simulink model "jerkControl2017"  (Simulink 8.9)
settings: Solver=FixedStepDiscrete  StartTime=0.0  StopTime="Config.SIMULATION_TIME "  FixedStep=Config.Ts  RelTol=1e-3  EnableMultiTasking=on
InitFcn:
  | %% initialize the simulation
  | cd(fileparts(which(bdroot)));
  | initJerkControl;
StopFcn:
  | %% stop the simulation
  | cd(fileparts(which(bdroot)));
  | stopJerkControl;
undefined symbols (not defined in the file or in its folder): Config, DiscIntNeverNeededParam, Gain, Reg, ROBOT_DOF, Sat, Sm
libraries: WBToolboxLibrary x69, simulink x4
(part 2 of 2)

== system jerkControl2017/emergency stop: joint limits/STOP IF THERE ARE SPIKES IN THE ENCODERS ==
  qj : Inport
  Enable : EnablePort
  Assertion : Assertion
  MATLAB Function : MATLAB Function  TreatAsAtomicUnit=on
  index1 : Constant  Value=Sat.maxJointsPositionDelta  VectorParams1D=off
  wires:
  qj/1 -> MATLAB Function/1(u)
  MATLAB Function/1(noSpikes) -> Assertion/1
  index1/1 -> MATLAB Function/2(delta_u_max)

== system jerkControl2017/synchronizer/GAZEBO_SYNCHRONIZER ==
  Enable : EnablePort
  Simulator Synchronizer : WBToolboxLibrary/Utilities/Simulator Synchronizer  period=Config.Ts  serverPortName='/clock/rpc'  clientPortName='/WBT_synchronizer/rpc:o'
      settings: SourceProductName=WholeBodyToolbox

== system jerkControl2017/synchronizer/REAL_TIME_SYNC ==
  Enable : EnablePort
  Real Time Synchronizer : WBToolboxLibrary/Utilities/Real Time Synchronizer  period=Config.Ts
      settings: SourceProductName=WholeBodyToolbox

== system jerkControl2017/Dump and visualize/Visualizer Forces and Momentum/dynamics_measured ==
  error : Inport
  Demux19 : Demux  Outputs=[3;3]
  Demux23 : Demux  Outputs=[6;6]
  Demux24 : Demux  Outputs=[3;3]
  left foot error wrench : Scope  NumInputPorts=2
  right foot error wrench : Scope  NumInputPorts=2
  wires:
  Demux19/2 -> right foot error wrench/2  "moments"
  Demux24/1 -> left foot error wrench/1  "forces"
  Demux24/2 -> left foot error wrench/2  "moments"
  Demux23/1 -> Demux24/1
  error/1 -> Demux23/1
  Demux19/1 -> right foot error wrench/1  "forces"
  Demux23/2 -> Demux19/1

== system jerkControl2017/Dump and visualize/Visualizer Forces and Momentum/star_dynamics ==
  error : Inport
  Demux19 : Demux  Outputs=[3;3]
  Demux23 : Demux  Outputs=[6;6]
  Demux24 : Demux  Outputs=[3;3]
  left foot error wrench : Scope  NumInputPorts=2
  right foot error wrench : Scope  NumInputPorts=2
  wires:
  Demux23/1 -> Demux24/1
  Demux19/1 -> right foot error wrench/1  "forces"
  Demux23/2 -> Demux19/1
  Demux19/2 -> right foot error wrench/2  "moments"
  Demux24/2 -> left foot error wrench/2  "moments"
  error/1 -> Demux23/1
  Demux24/1 -> left foot error wrench/1  "forces"

== system jerkControl2017/Dump and visualize/Visualizer Forces and Momentum/star_measured ==
  error : Inport
  Demux19 : Demux  Outputs=[3;3]
  Demux23 : Demux  Outputs=[6;6]
  Demux24 : Demux  Outputs=[3;3]
  left foot error wrench : Scope  NumInputPorts=2
  right foot error wrench : Scope  NumInputPorts=2
  wires:
  Demux19/2 -> right foot error wrench/2  "moments"
  Demux24/1 -> left foot error wrench/1  "forces"
  Demux24/2 -> left foot error wrench/2  "moments"
  Demux23/1 -> Demux24/1
  error/1 -> Demux23/1
  Demux19/1 -> right foot error wrench/1  "forces"
  Demux23/2 -> Demux19/1

== system jerkControl2017/Dynamics and Kinematics/Dynamics/Add motors reflected inertia ==
  M : Inport
  Add motor reflected inertias : MATLAB Function  TreatAsAtomicUnit=on
  Constant : Constant  Value=Config.USE_MOTOR_REFLECTED_INERTIA
  Switch : Switch  Criteria=u2 > Threshold
  M_with_motor_inertia : Outport
  wires:
  M/1 -> Switch/3, Add motor reflected inertias/1(M)
  Constant/1 -> Switch/2
  Add motor reflected inertias/1(M_with_inertia) -> Switch/1
  Switch/1 -> M_with_motor_inertia/1

== system jerkControl2017/Dynamics and Kinematics/Kinematics/xCom ==
  w_H_b : Inport
  qj : Inport  Port=2
  CoM : WBToolboxLibrary/Model/Kinematics/ForwardKinematics  frameName=Frames.COM
      settings: SourceProductName=WholeBodyToolbox
  "CoM6D ->  CoMXYZ2" : Selector  NumberOfDimensions=2  InputPortWidth=7  IndexOptions=Index vector (dialog),Index vector (dialog)  Indices=[1 2 3],[4]  OutputSizes=1,1
  xCoM : Outport
  wires:
  qj/1 -> CoM/2
  "CoM6D ->  CoMXYZ2"/1 -> xCoM/1
  CoM/1 -> "CoM6D ->  CoMXYZ2"/1
  w_H_b/1 -> CoM/1

== system jerkControl2017/Jerk Control/Compute angular momentum integral error (YOGA)/Compute base to fixed link transform ==
  jointPos : Inport
  Constant7 : Constant  Value=eye(4)
  "inv  " : Product  Inputs=/  Multiplication=Matrix(*)
  inv  1 : Product  Inputs=/  Multiplication=Matrix(*)
  l_sole to root_link relative transform : WBToolboxLibrary/Model/Kinematics/ForwardKinematics  frameName=Frames.LEFT_FOOT
      settings: SourceProductName=WholeBodyToolbox
  r_sole to root_link relative transform : WBToolboxLibrary/Model/Kinematics/ForwardKinematics  frameName=Frames.RIGHT_FOOT
      settings: SourceProductName=WholeBodyToolbox
  fixed_l_sole_H_b : Outport
  fixed_r_sole_H_b : Outport  Port=2
  wires:
  Constant7/1 -> l_sole to root_link relative transform/1, r_sole to root_link relative transform/1
  inv  1/1 -> fixed_r_sole_H_b/1
  "inv  "/1 -> fixed_l_sole_H_b/1
  jointPos/1 -> r_sole to root_link relative transform/2, l_sole to root_link relative transform/2
  l_sole to root_link relative transform/1 -> "inv  "/1
  r_sole to root_link relative transform/1 -> inv  1/1

== system jerkControl2017/Jerk Control/Estimate Contact Forces and Parametrization/From body to Mixed Representation ==
  w_H_l_sole : Inport
  w_H_r_sole : Inport  Port=2
  contactForces_wbd : Inport  Port=3
  MATLAB Function : MATLAB Function  TreatAsAtomicUnit=on
  contactForces_est : Outport
  wires:
  w_H_l_sole/1 -> MATLAB Function/1(w_H_l_sole)
  w_H_r_sole/1 -> MATLAB Function/2(w_H_r_sole)
  contactForces_wbd/1 -> MATLAB Function/3(f_body)
  MATLAB Function/1(f_mixed) -> contactForces_est/1

== system jerkControl2017/Jerk Control/Estimate Contact Forces and Parametrization/Get Parametrization from Forces ==
  LEFT_RIGHT_FOOT_IN_CONTACT : Inport
  contactForces_est : Inport  Port=2
  Constant : Constant  Value=[0;0;Config.fZmin;0;0;0]
  Constant1 : Constant  Value=[0;0;Config.fZmin;0;0;0]
  Demux : Demux  Outputs=[6;6]
  Demux1 : Demux  Outputs=[1;1]
  MATLAB Function1 : MATLAB Function  TreatAsAtomicUnit=on
  MATLAB Function2 : MATLAB Function  TreatAsAtomicUnit=on
  MatrixMultiply : Product
  MatrixMultiply1 : Product
  Mux : Mux  Inputs=2
  Switch : Switch  Criteria=u2 > Threshold
  Switch1 : Switch  Criteria=u2 > Threshold
  xi : Outport
  tag scope: xi_LFoot=global, xi_RFoot=global
  wires:
  Mux/1 -> xi/1
  contactForces_est/1 -> Demux/1
  LEFT_RIGHT_FOOT_IN_CONTACT/1 -> Demux1/1
  MATLAB Function1/1(xi) -> MatrixMultiply1/1
  MATLAB Function2/1(xi) -> MatrixMultiply/1
  Demux1/1 -> Switch/2, MatrixMultiply1/2
  Demux1/2 -> Switch1/2, MatrixMultiply/2
  MatrixMultiply1/1 -> Mux/1, [xi_LFoot]
  MatrixMultiply/1 -> Mux/2, [xi_RFoot]
  Demux/1 -> Switch/1
  Constant/1 -> Switch/3
  Demux/2 -> Switch1/1
  Constant1/1 -> Switch1/3
  Switch1/1 -> MATLAB Function2/1(contactForces)
  Switch/1 -> MATLAB Function1/1(contactForces)

== system jerkControl2017/Jerk Control/Integrate the Input Contact Forces Param. Derivative/Demux xiDot ==
  xiDot_star : Inport
  LEFT_RIGHT_FOOT_IN_CONTACT : Inport  Port=2
  M : Inport  Port=3
  Compute Initial Conditions LFoot : Subsystem
  Compute Initial Conditions RFoot : Subsystem
  Demux : Demux  Outputs=[6;6]
  Demux1 : Demux  Outputs=[1;1]
  MATLAB Function1 : MATLAB Function  TreatAsAtomicUnit=on
  MATLAB Function2 : MATLAB Function  TreatAsAtomicUnit=on
  xiDot_LFoot : Outport
  LFootContactActivation : Outport  Port=2
  init_xi_LFoot : Outport  Port=3
  xiDot_RFoot : Outport  Port=4
  RFootContactActivation : Outport  Port=5
  init_xi_RFoot : Outport  Port=6
  wires:
  Demux/2 -> xiDot_RFoot/1
  xiDot_star/1 -> Demux/1
  LEFT_RIGHT_FOOT_IN_CONTACT/1 -> Demux1/1
  Demux/1 -> xiDot_LFoot/1
  Demux1/1 -> Compute Initial Conditions LFoot/1(FOOT_IS_IN_CONTACT), LFootContactActivation/1
  Demux1/2 -> Compute Initial Conditions RFoot/1(FOOT_IS_IN_CONTACT), RFootContactActivation/1
  M/1 -> Compute Initial Conditions RFoot/2(M), Compute Initial Conditions LFoot/2(M)
  Compute Initial Conditions LFoot/1(contactForcesOneFoot_0) -> MATLAB Function1/1(contactForces)
  Compute Initial Conditions RFoot/1(contactForcesOneFoot_0) -> MATLAB Function2/1(contactForces)
  MATLAB Function1/1(xi) -> init_xi_LFoot/1
  MATLAB Function2/1(xi) -> init_xi_RFoot/1

== system jerkControl2017/Jerk Control/Integrate the Input Contact Forces Param. Derivative/From Parametrization to Forces ==
  LFootContactActivation : Inport
  xi_LFoot : Inport  Port=2
  xi_RFoot : Inport  Port=3
  RFootContactActivation : Inport  Port=4
  MATLAB Function : MATLAB Function  TreatAsAtomicUnit=on
  MATLAB Function1 : MATLAB Function  TreatAsAtomicUnit=on
  MatrixMultiply1 : Product
  MatrixMultiply2 : Product
  contactForces_LFoot : Outport
  contactForces_RFoot : Outport  Port=2
  wires:
  MatrixMultiply1/1 -> contactForces_LFoot/1
  MATLAB Function/1(contactForces) -> MatrixMultiply1/2
  MATLAB Function1/1(contactForces) -> MatrixMultiply2/2
  MatrixMultiply2/1 -> contactForces_RFoot/1
  LFootContactActivation/1 -> MatrixMultiply1/1
  xi_LFoot/1 -> MATLAB Function/1(xi)
  RFootContactActivation/1 -> MatrixMultiply2/1
  xi_RFoot/1 -> MATLAB Function1/1(xi)

== system jerkControl2017/Jerk Control/Integrate the Input Contact Forces Param. Derivative/deadZone ==
  u : Inport
  Constant : Constant  Value=Sat.deadZoneThreshold
  MATLAB Function : MATLAB Function  TreatAsAtomicUnit=on
  u_cut : Outport
  wires:
  MATLAB Function/1(y) -> u_cut/1
  u/1 -> MATLAB Function/1(u)
  Constant/1 -> MATLAB Function/2(thr)

== system jerkControl2017/Robot State and References/Internal Coordinator/Base to fixed_link ==
  qj : Inport
  inertial : Inport  Port=2
  Constant1 : Constant  Value=Config.LEFT_FOOT_IN_CONTACT_AT_0
  Constant7 : Constant  Value=eye(4)
  LFoot to world transform (fixed base) : WBToolboxLibrary/Model/Kinematics/ForwardKinematics  frameName=Frames.LEFT_FOOT
      settings: SourceProductName=WholeBodyToolbox
  RFoot to world transform (fixed base) : WBToolboxLibrary/Model/Kinematics/ForwardKinematics  frameName=Frames.RIGHT_FOOT
      settings: SourceProductName=WholeBodyToolbox
  Switch : Switch  Criteria=u2 > Threshold
  "fixedFoot to base link transform " : Subsystem
  fixed_LFoot_H_b : Outport
  wires:
  "fixedFoot to base link transform "/1(link_H_b) -> fixed_LFoot_H_b/1
  inertial/1 -> "fixedFoot to base link transform "/2(inertial)
  qj/1 -> "fixedFoot to base link transform "/1(qj), RFoot to world transform (fixed base)/2, LFoot to world transform (fixed base)/2
  Constant7/1 -> LFoot to world transform (fixed base)/1, RFoot to world transform (fixed base)/1, "fixedFoot to base link transform "/4(w_H_base_fixed)
  Switch/1 -> "fixedFoot to base link transform "/3(w_H_link)
  LFoot to world transform (fixed base)/1 -> Switch/1
  RFoot to world transform (fixed base)/1 -> Switch/3
  Constant1/1 -> Switch/2

== system jerkControl2017/Robot State and References/Internal Coordinator/Compute State Velocity ==
  qj : Inport
  w_H_b : Inport  Port=2
  "feetInContact " : Inport  Port=3
  Compute Base Velocity : MATLAB Function  TreatAsAtomicUnit=on
  Feet Jacobians : Subsystem
  GetMeasurement : WBToolboxLibrary/States/GetMeasurement  measuredType=Joints Velocity
      settings: SourceProductName=WholeBodyToolbox
  Mux : Mux  Inputs=2
  nu : Outport
  wires:
  GetMeasurement/1 -> Mux/2, Compute Base Velocity/4(jointVel)
  Mux/1 -> nu/1
  "feetInContact "/1 -> Compute Base Velocity/3(feetContactStatus)
  qj/1 -> Feet Jacobians/1(qj)
  w_H_b/1 -> Feet Jacobians/2(w_H_b)
  Feet Jacobians/1(J_LFoot) -> Compute Base Velocity/1(J_l_sole)
  Feet Jacobians/2(J_RFoot) -> Compute Base Velocity/2(J_r_sole)
  Compute Base Velocity/1(nu_b) -> Mux/1

== system jerkControl2017/Robot State and References/Internal Coordinator/xCom ==
  w_H_b : Inport
  qj : Inport  Port=2
  CoM : WBToolboxLibrary/Model/Kinematics/ForwardKinematics  frameName=Frames.COM
      settings: SourceProductName=WholeBodyToolbox
  "CoM6D ->  CoMXYZ2" : Selector  NumberOfDimensions=2  InputPortWidth=7  IndexOptions=Index vector (dialog),Index vector (dialog)  Indices=[1 2 3],[4]  OutputSizes=1,1
  xCoM : Outport
  wires:
  qj/1 -> CoM/2
  "CoM6D ->  CoMXYZ2"/1 -> xCoM/1
  CoM/1 -> "CoM6D ->  CoMXYZ2"/1
  w_H_b/1 -> CoM/1

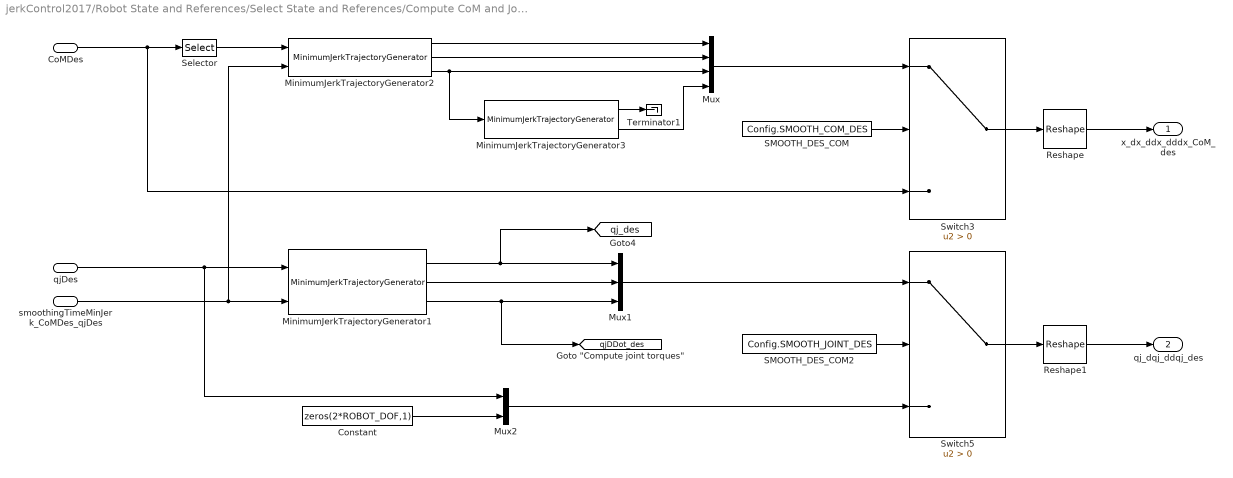
== system jerkControl2017/Robot State and References/Select State and References/Compute CoM and Joint References ==
  CoMDes : Inport
  qjDes : Inport  Port=2
  smoothingTimeMinJerk_CoMDes_qjDes : Inport  Port=3
  Constant : Constant  Value=zeros(2*ROBOT_DOF,1)
  MinimumJerkTrajectoryGenerator1 : WBToolboxLibrary/Utilities/MinimumJerkTrajectoryGenerator  externalSettlingTime=on  settlingTime=0.01  sampleTime=Config.Ts  resetOnSettlingTime=off  firstDerivatives=on  secondDerivatives=on  explicitInitialValue=off
      settings: SourceProductName=WholeBodyToolbox
  MinimumJerkTrajectoryGenerator2 : WBToolboxLibrary/Utilities/MinimumJerkTrajectoryGenerator  externalSettlingTime=on  settlingTime=0.01  sampleTime=Config.Ts  resetOnSettlingTime=off  firstDerivatives=on  secondDerivatives=on  explicitInitialValue=off
      settings: SourceProductName=WholeBodyToolbox
  MinimumJerkTrajectoryGenerator3 : WBToolboxLibrary/Utilities/MinimumJerkTrajectoryGenerator  externalSettlingTime=off  settlingTime=0.005  sampleTime=Config.Ts  resetOnSettlingTime=off  firstDerivatives=on  secondDerivatives=off  explicitInitialValue=off
      settings: SourceProductName=WholeBodyToolbox
  Mux : Mux
  Mux1 : Mux  Inputs=3
  Mux2 : Mux  Inputs=2
  Reshape : Reshape  OutputDimensionality=Customize  OutputDimensions=[3,4]
  Reshape1 : Reshape  OutputDimensionality=Customize  OutputDimensions=[ROBOT_DOF,3]
  SMOOTH_DES_COM : Constant  Value=Config.SMOOTH_COM_DES
  SMOOTH_DES_COM2 : Constant  Value=Config.SMOOTH_JOINT_DES
  Selector : Selector  InputPortWidth=12  IndexOptions=Index vector (dialog)  Indices=[1 2 3]  OutputSizes=1
  Switch3 : Switch  Criteria=u2 > Threshold
  Switch5 : Switch  Criteria=u2 > Threshold
  Terminator1 : Terminator
  x_dx_ddx_dddx_CoM_des : Outport
  qj_dqj_ddqj_des : Outport  Port=2
  tag scope: qjDDot_des=global, qj_des=global
  wires:
  MinimumJerkTrajectoryGenerator1/2 -> Mux1/2
  SMOOTH_DES_COM2/1 -> Switch5/2
  Selector/1 -> MinimumJerkTrajectoryGenerator2/1
  MinimumJerkTrajectoryGenerator2/2 -> Mux/2
  qjDes/1 -> Mux2/1, MinimumJerkTrajectoryGenerator1/1
  smoothingTimeMinJerk_CoMDes_qjDes/1 -> MinimumJerkTrajectoryGenerator2/2, MinimumJerkTrajectoryGenerator1/2
  SMOOTH_DES_COM/1 -> Switch3/2
  Switch5/1 -> Reshape1/1
  Mux/1 -> Switch3/1
  Switch3/1 -> Reshape/1
  MinimumJerkTrajectoryGenerator2/1 -> Mux/1
  Reshape/1 -> x_dx_ddx_dddx_CoM_des/1
  MinimumJerkTrajectoryGenerator3/1 -> Terminator1/1
  Mux1/1 -> Switch5/1
  Reshape1/1 -> qj_dqj_ddqj_des/1
  CoMDes/1 -> Switch3/3, Selector/1
  Constant/1 -> Mux2/2
  Mux2/1 -> Switch5/3
  MinimumJerkTrajectoryGenerator1/1 -> [qj_des], Mux1/1
  MinimumJerkTrajectoryGenerator1/3 -> Mux1/3, [qjDDot_des]
  MinimumJerkTrajectoryGenerator3/2 -> Mux/4
  MinimumJerkTrajectoryGenerator2/3 -> Mux/3, MinimumJerkTrajectoryGenerator3/1

== system jerkControl2017/Robot State and References/State Machine Yoga/Compute State Velocity ==
  qj : Inport
  w_H_b : Inport  Port=2
  "feetInContact " : Inport  Port=3
  Compute Base Velocity : MATLAB Function  TreatAsAtomicUnit=on
  Feet Jacobians : Subsystem
  GetMeasurement : WBToolboxLibrary/States/GetMeasurement  measuredType=Joints Velocity
      settings: SourceProductName=WholeBodyToolbox
  Mux : Mux  Inputs=2
  nu : Outport
  wires:
  Mux/1 -> nu/1
  Compute Base Velocity/1(nu_b) -> Mux/1
  qj/1 -> Feet Jacobians/1(qj)
  w_H_b/1 -> Feet Jacobians/2(w_H_b)
  Feet Jacobians/1(J_LFoot) -> Compute Base Velocity/1(J_l_sole)
  Feet Jacobians/2(J_RFoot) -> Compute Base Velocity/2(J_r_sole)
  "feetInContact "/1 -> Compute Base Velocity/3(feetContactStatus)
  GetMeasurement/1 -> Compute Base Velocity/4(jointVel), Mux/2

== system jerkControl2017/Robot State and References/State Machine Yoga/Compute base to fixed link transform ==
  qj : Inport
  inertial : Inport  Port=2
  Constant7 : Constant  Value=eye(4)
  LFoot to world transform (fixed base) : WBToolboxLibrary/Model/Kinematics/ForwardKinematics  frameName=Frames.LEFT_FOOT
      settings: SourceProductName=WholeBodyToolbox
  RFoot to world transform (fixed base) : WBToolboxLibrary/Model/Kinematics/ForwardKinematics  frameName=Frames.RIGHT_FOOT
      settings: SourceProductName=WholeBodyToolbox
  "fixedLFoot to base link transform " : Subsystem
  fixedRFoot to base link transform : Subsystem
  fixed_LFoot_H_b : Outport
  fixed_RFoot_H_b : Outport  Port=2
  wires:
  Constant7/1 -> fixedRFoot to base link transform/4(w_H_base_fixed), "fixedLFoot to base link transform "/4(w_H_base_fixed), RFoot to world transform (fixed base)/1, LFoot to world transform (fixed base)/1
  fixedRFoot to base link transform/1(link_H_b) -> fixed_RFoot_H_b/1
  "fixedLFoot to base link transform "/1(link_H_b) -> fixed_LFoot_H_b/1
  LFoot to world transform (fixed base)/1 -> "fixedLFoot to base link transform "/3(w_H_link)
  RFoot to world transform (fixed base)/1 -> fixedRFoot to base link transform/3(w_H_link)
  qj/1 -> fixedRFoot to base link transform/1(qj), "fixedLFoot to base link transform "/1(qj), RFoot to world transform (fixed base)/2, LFoot to world transform (fixed base)/2
  inertial/1 -> fixedRFoot to base link transform/2(inertial), "fixedLFoot to base link transform "/2(inertial)

== system jerkControl2017/Robot State and References/State Machine Yoga/xCom ==
  w_H_b : Inport
  qj : Inport  Port=2
  CoM : WBToolboxLibrary/Model/Kinematics/ForwardKinematics  frameName=Frames.COM
      settings: SourceProductName=WholeBodyToolbox
  "CoM6D ->  CoMXYZ2" : Selector  NumberOfDimensions=2  InputPortWidth=7  IndexOptions=Index vector (dialog),Index vector (dialog)  Indices=[1 2 3],[4]  OutputSizes=1,1
  xCoM : Outport
  wires:
  qj/1 -> CoM/2
  "CoM6D ->  CoMXYZ2"/1 -> xCoM/1
  CoM/1 -> "CoM6D ->  CoMXYZ2"/1
  w_H_b/1 -> CoM/1

== system jerkControl2017/Robot State and References/State Machine Yoga/xCom1 ==
  w_H_b : Inport
  qj : Inport  Port=2
  CoM : WBToolboxLibrary/Model/Kinematics/ForwardKinematics  frameName=Frames.COM
      settings: SourceProductName=WholeBodyToolbox
  "CoM6D ->  CoMXYZ2" : Selector  NumberOfDimensions=2  InputPortWidth=7  IndexOptions=Index vector (dialog),Index vector (dialog)  Indices=[1 2 3],[4]  OutputSizes=1,1
  xCoM : Outport
  wires:
  qj/1 -> CoM/2
  "CoM6D ->  CoMXYZ2"/1 -> xCoM/1
  CoM/1 -> "CoM6D ->  CoMXYZ2"/1
  w_H_b/1 -> CoM/1

== system jerkControl2017/Jerk Control/Integrate the Input Contact Forces Param. Derivative/Demux xiDot/Compute Initial Conditions LFoot ==
  FOOT_IS_IN_CONTACT : Inport
  M : Inport  Port=2
  Check Previous Foot_in_contact : MATLAB Function  TreatAsAtomicUnit=on
  Constant : Constant  Value=[0; 0; Sm.wrench_thresholdContactOn; 0; 0; 0]
  Gain : Gain  Gain=[0; 0; 0.5.*Config.GRAVITY_ACC; 0; 0; 0]
  Selector : Selector  NumberOfDimensions=2  InputPortWidth=3  IndexOptions=Index vector (dialog),Index vector (dialog)  Indices=1,1  OutputSizes=1,1
  Switch : Switch  Criteria=u2 > Threshold  Threshold=0.5
  contactForcesOneFoot_0 : Outport
  wires:
  M/1 -> Selector/1
  Selector/1 -> Gain/1
  Switch/1 -> contactForcesOneFoot_0/1
  Gain/1 -> Switch/1  "initial contact forces while balancing"
  Constant/1 -> Switch/3  "initial contact forces after balancing on the other foot"
  FOOT_IS_IN_CONTACT/1 -> Check Previous Foot_in_contact/1(currentFootInContact)
  Check Previous Foot_in_contact/1(prevFootBoolean) -> Switch/2

== system jerkControl2017/Jerk Control/Integrate the Input Contact Forces Param. Derivative/Demux xiDot/Compute Initial Conditions RFoot ==
  FOOT_IS_IN_CONTACT : Inport
  M : Inport  Port=2
  Check Previous Foot_in_contact : MATLAB Function  TreatAsAtomicUnit=on
  Constant : Constant  Value=[0; 0; Sm.wrench_thresholdContactOn; 0; 0; 0]
  Gain : Gain  Gain=[0; 0; 0.5.*Config.GRAVITY_ACC; 0; 0; 0]
  Selector : Selector  NumberOfDimensions=2  InputPortWidth=3  IndexOptions=Index vector (dialog),Index vector (dialog)  Indices=1,1  OutputSizes=1,1
  Switch : Switch  Criteria=u2 > Threshold  Threshold=0.5
  contactForcesOneFoot_0 : Outport
  wires:
  M/1 -> Selector/1
  Selector/1 -> Gain/1
  Switch/1 -> contactForcesOneFoot_0/1
  Gain/1 -> Switch/1  "initial contact forces while balancing"
  Constant/1 -> Switch/3  "initial contact forces after balancing on the other foot"
  FOOT_IS_IN_CONTACT/1 -> Check Previous Foot_in_contact/1(currentFootInContact)
  Check Previous Foot_in_contact/1(prevFootBoolean) -> Switch/2

== system jerkControl2017/Robot State and References/Internal Coordinator/Base to fixed_link/fixedFoot to base link transform  ==
  qj : Inport
  inertial : Inport  Port=2
  w_H_link : Inport  Port=3
  w_H_base_fixed : Inport  Port=4
  Fixed base to imu transform : WBToolboxLibrary/Model/Kinematics/ForwardKinematics  frameName=Frames.IMU
      settings: SourceProductName=WholeBodyToolbox
  Fixed base to root link transform : WBToolboxLibrary/Model/Kinematics/ForwardKinematics  frameName=Frames.BASE
      settings: SourceProductName=WholeBodyToolbox
  Inv\* : Product  Inputs=/*  Multiplication=Matrix(*)
  "Inv\\*  " : Product  Inputs=/*  Multiplication=Matrix(*)
  Neck Position : WBToolboxLibrary/Utilities/YarpRead  portName=Ports.NECK_POS  signalSize=Ports.NECK_POS_PORT_SIZE  timeout=0.5  blocking=off  timestamp=off  autoconnect=on  errorOnConnection=off
      settings: SourceProductName=WholeBodyToolbox
  Selector1 : Selector  InputPortWidth=Ports.IMU_PORT_SIZE  IndexOptions=Index vector (dialog)  Indices=Ports.IMU_PORT_ORIENTATION_INDEX  OutputSizes=1
  Selector2 : Selector  InputPortWidth=Ports.IMU_PORT_SIZE  IndexOptions=Index vector (dialog)  Indices=Ports.IMU_PORT_ORIENTATION_INDEX  OutputSizes=1
  Switch6 : Switch  Criteria=u2 > Threshold
  USE_IMU4EST_BASE : Constant  Value=Config.USE_IMU4EST_BASE
  fromImuToHomogeousTransformFCN : MATLAB Function  TreatAsAtomicUnit=on
  holder 1 : WBToolboxLibrary/Utilities/holder 
      settings: SourceProductName=WholeBodyToolbox
  holder 2 : WBToolboxLibrary/Utilities/holder 
      settings: SourceProductName=WholeBodyToolbox
  neck transform : Subsystem
  link_H_b : Outport
  wires:
  Switch6/1 -> link_H_b/1
  "Inv\\*  "/1 -> Switch6/3, fromImuToHomogeousTransformFCN/3(fixedLink_H_base)  "link_H_root"
  USE_IMU4EST_BASE/1 -> Switch6/2
  Inv\*/1 -> fromImuToHomogeousTransformFCN/1(imu_H_fixedLink), holder 1/1  "imu_H_link"
  holder 2/1 -> Selector2/1
  Fixed base to imu transform/1 -> Inv\*/1
  holder 1/1 -> fromImuToHomogeousTransformFCN/2(imu_H_fixedLink_0)
  qj/1 -> Fixed base to imu transform/2, Fixed base to root link transform/2
  fromImuToHomogeousTransformFCN/1(w_H_b) -> Switch6/1
  Fixed base to root link transform/1 -> "Inv\\*  "/2
  inertial/1 -> holder 2/1, Selector1/1
  Neck Position/1 -> neck transform/1(neck port)
  neck transform/1(neck position) -> fromImuToHomogeousTransformFCN/6(neck_pos)
  w_H_link/1 -> "Inv\\*  "/1, Inv\*/2
  w_H_base_fixed/1 -> Fixed base to root link transform/1, Fixed base to imu transform/1
  Selector2/1 -> fromImuToHomogeousTransformFCN/4(rpyFromIMU_0)
  Selector1/1 -> fromImuToHomogeousTransformFCN/5(rpyFromIMU)

== system jerkControl2017/Robot State and References/Internal Coordinator/Compute State Velocity/Feet Jacobians ==
  qj : Inport
  w_H_b : Inport  Port=2
  Jacobian LFoot : WBToolboxLibrary/Model/Jacobians/Jacobian  frameName=Frames.LEFT_FOOT
      settings: SourceProductName=WholeBodyToolbox
  Jacobian RFoot : WBToolboxLibrary/Model/Jacobians/Jacobian  frameName=Frames.RIGHT_FOOT
      settings: SourceProductName=WholeBodyToolbox
  J_LFoot : Outport
  J_RFoot : Outport  Port=2
  wires:
  Jacobian LFoot/1 -> J_LFoot/1
  Jacobian RFoot/1 -> J_RFoot/1
  w_H_b/1 -> Jacobian RFoot/1, Jacobian LFoot/1
  qj/1 -> Jacobian LFoot/2, Jacobian RFoot/2

== system jerkControl2017/Robot State and References/State Machine Yoga/Compute State Velocity/Feet Jacobians ==
  qj : Inport
  w_H_b : Inport  Port=2
  Jacobian LFoot : WBToolboxLibrary/Model/Jacobians/Jacobian  frameName=Frames.LEFT_FOOT
      settings: SourceProductName=WholeBodyToolbox
  Jacobian RFoot : WBToolboxLibrary/Model/Jacobians/Jacobian  frameName=Frames.RIGHT_FOOT
      settings: SourceProductName=WholeBodyToolbox
  J_LFoot : Outport
  J_RFoot : Outport  Port=2
  wires:
  Jacobian LFoot/1 -> J_LFoot/1
  Jacobian RFoot/1 -> J_RFoot/1
  w_H_b/1 -> Jacobian RFoot/1, Jacobian LFoot/1
  qj/1 -> Jacobian LFoot/2, Jacobian RFoot/2

== system jerkControl2017/Robot State and References/State Machine Yoga/Compute base to fixed link transform/fixedLFoot to base link transform  ==
  qj : Inport
  inertial : Inport  Port=2
  w_H_link : Inport  Port=3
  w_H_base_fixed : Inport  Port=4
  Fixed base to imu transform : WBToolboxLibrary/Model/Kinematics/ForwardKinematics  frameName=Frames.IMU
      settings: SourceProductName=WholeBodyToolbox
  Fixed base to root link transform : WBToolboxLibrary/Model/Kinematics/ForwardKinematics  frameName=Frames.BASE
      settings: SourceProductName=WholeBodyToolbox
  Inv\* : Product  Inputs=/*  Multiplication=Matrix(*)
  "Inv\\*  " : Product  Inputs=/*  Multiplication=Matrix(*)
  Neck Position : WBToolboxLibrary/Utilities/YarpRead  portName=Ports.NECK_POS  signalSize=Ports.NECK_POS_PORT_SIZE  timeout=0.5  blocking=off  timestamp=off  autoconnect=on  errorOnConnection=off
      settings: SourceProductName=WholeBodyToolbox
  Selector1 : Selector  InputPortWidth=Ports.IMU_PORT_SIZE  IndexOptions=Index vector (dialog)  Indices=Ports.IMU_PORT_ORIENTATION_INDEX  OutputSizes=1
  Selector2 : Selector  InputPortWidth=Ports.IMU_PORT_SIZE  IndexOptions=Index vector (dialog)  Indices=Ports.IMU_PORT_ORIENTATION_INDEX  OutputSizes=1
  Switch6 : Switch  Criteria=u2 > Threshold
  USE_IMU4EST_BASE : Constant  Value=Config.USE_IMU4EST_BASE
  fromImuToHomogeousTransformFCN : MATLAB Function  TreatAsAtomicUnit=on
  holder 1 : WBToolboxLibrary/Utilities/holder 
      settings: SourceProductName=WholeBodyToolbox
  holder 2 : WBToolboxLibrary/Utilities/holder 
      settings: SourceProductName=WholeBodyToolbox
  neck transform : Subsystem
  link_H_b : Outport
  wires:
  Switch6/1 -> link_H_b/1
  "Inv\\*  "/1 -> Switch6/3, fromImuToHomogeousTransformFCN/3(fixedLink_H_base)  "link_H_root"
  USE_IMU4EST_BASE/1 -> Switch6/2
  Inv\*/1 -> fromImuToHomogeousTransformFCN/1(imu_H_fixedLink), holder 1/1  "imu_H_link"
  holder 2/1 -> Selector2/1
  Fixed base to imu transform/1 -> Inv\*/1
  holder 1/1 -> fromImuToHomogeousTransformFCN/2(imu_H_fixedLink_0)
  qj/1 -> Fixed base to imu transform/2, Fixed base to root link transform/2
  fromImuToHomogeousTransformFCN/1(w_H_b) -> Switch6/1
  Fixed base to root link transform/1 -> "Inv\\*  "/2
  inertial/1 -> holder 2/1, Selector1/1
  Neck Position/1 -> neck transform/1(neck port)
  neck transform/1(neck position) -> fromImuToHomogeousTransformFCN/6(neck_pos)
  w_H_link/1 -> "Inv\\*  "/1, Inv\*/2
  w_H_base_fixed/1 -> Fixed base to root link transform/1, Fixed base to imu transform/1
  Selector2/1 -> fromImuToHomogeousTransformFCN/4(rpyFromIMU_0)
  Selector1/1 -> fromImuToHomogeousTransformFCN/5(rpyFromIMU)

== system jerkControl2017/Robot State and References/State Machine Yoga/Compute base to fixed link transform/fixedRFoot to base link transform ==
  qj : Inport
  inertial : Inport  Port=2
  w_H_link : Inport  Port=3
  w_H_base_fixed : Inport  Port=4
  Fixed base to imu transform : WBToolboxLibrary/Model/Kinematics/ForwardKinematics  frameName=Frames.IMU
      settings: SourceProductName=WholeBodyToolbox
  Fixed base to root link transform : WBToolboxLibrary/Model/Kinematics/ForwardKinematics  frameName=Frames.BASE
      settings: SourceProductName=WholeBodyToolbox
  Inv\* : Product  Inputs=/*  Multiplication=Matrix(*)
  "Inv\\*  " : Product  Inputs=/*  Multiplication=Matrix(*)
  Neck Position : WBToolboxLibrary/Utilities/YarpRead  portName=Ports.NECK_POS  signalSize=Ports.NECK_POS_PORT_SIZE  timeout=0.5  blocking=off  timestamp=off  autoconnect=on  errorOnConnection=off
      settings: SourceProductName=WholeBodyToolbox
  Selector1 : Selector  InputPortWidth=Ports.IMU_PORT_SIZE  IndexOptions=Index vector (dialog)  Indices=Ports.IMU_PORT_ORIENTATION_INDEX  OutputSizes=1
  Selector2 : Selector  InputPortWidth=Ports.IMU_PORT_SIZE  IndexOptions=Index vector (dialog)  Indices=Ports.IMU_PORT_ORIENTATION_INDEX  OutputSizes=1
  Switch6 : Switch  Criteria=u2 > Threshold
  USE_IMU4EST_BASE : Constant  Value=Config.USE_IMU4EST_BASE
  fromImuToHomogeousTransformFCN : MATLAB Function  TreatAsAtomicUnit=on
  holder 1 : WBToolboxLibrary/Utilities/holder 
      settings: SourceProductName=WholeBodyToolbox
  holder 2 : WBToolboxLibrary/Utilities/holder 
      settings: SourceProductName=WholeBodyToolbox
  neck transform : Subsystem
  link_H_b : Outport
  wires:
  Switch6/1 -> link_H_b/1
  "Inv\\*  "/1 -> Switch6/3, fromImuToHomogeousTransformFCN/3(fixedLink_H_base)  "link_H_root"
  USE_IMU4EST_BASE/1 -> Switch6/2
  Inv\*/1 -> fromImuToHomogeousTransformFCN/1(imu_H_fixedLink), holder 1/1  "imu_H_link"
  holder 2/1 -> Selector2/1
  Fixed base to imu transform/1 -> Inv\*/1
  holder 1/1 -> fromImuToHomogeousTransformFCN/2(imu_H_fixedLink_0)
  qj/1 -> Fixed base to imu transform/2, Fixed base to root link transform/2
  fromImuToHomogeousTransformFCN/1(w_H_b) -> Switch6/1
  Fixed base to root link transform/1 -> "Inv\\*  "/2
  inertial/1 -> holder 2/1, Selector1/1
  Neck Position/1 -> neck transform/1(neck port)
  neck transform/1(neck position) -> fromImuToHomogeousTransformFCN/6(neck_pos)
  w_H_link/1 -> "Inv\\*  "/1, Inv\*/2
  w_H_base_fixed/1 -> Fixed base to root link transform/1, Fixed base to imu transform/1
  Selector2/1 -> fromImuToHomogeousTransformFCN/4(rpyFromIMU_0)
  Selector1/1 -> fromImuToHomogeousTransformFCN/5(rpyFromIMU)

== system jerkControl2017/Robot State and References/Internal Coordinator/Base to fixed_link/fixedFoot to base link transform /neck transform ==
  neck port : Inport
  Constant : Constant  Value=zeros(3,1)
  Gain : Gain  Gain=pi/180
  Selector1 : Selector  InputPortWidth=Ports.NECK_POS_PORT_SIZE  IndexOptions=Index vector (dialog)  Indices=[1:3]  OutputSizes=1
  Switch : Switch  Criteria=u2 > Threshold
  USE_IMU4EST_BASE1 : Constant  Value=Config.CORRECT_NECK_IMU
  neck position : Outport
  wires:
  neck port/1 -> Gain/1
  USE_IMU4EST_BASE1/1 -> Switch/2
  Switch/1 -> neck position/1
  Gain/1 -> Selector1/1
  Constant/1 -> Switch/3
  Selector1/1 -> Switch/1  "neck pos"

== system jerkControl2017/Robot State and References/State Machine Yoga/Compute base to fixed link transform/fixedLFoot to base link transform /neck transform ==
  neck port : Inport
  Constant : Constant  Value=zeros(3,1)
  Gain : Gain  Gain=pi/180
  Selector1 : Selector  InputPortWidth=Ports.NECK_POS_PORT_SIZE  IndexOptions=Index vector (dialog)  Indices=[1:3]  OutputSizes=1
  Switch : Switch  Criteria=u2 > Threshold
  USE_IMU4EST_BASE1 : Constant  Value=Config.CORRECT_NECK_IMU
  neck position : Outport
  wires:
  neck port/1 -> Gain/1
  USE_IMU4EST_BASE1/1 -> Switch/2
  Switch/1 -> neck position/1
  Gain/1 -> Selector1/1
  Constant/1 -> Switch/3
  Selector1/1 -> Switch/1  "neck pos"

== system jerkControl2017/Robot State and References/State Machine Yoga/Compute base to fixed link transform/fixedRFoot to base link transform/neck transform ==
  neck port : Inport
  Constant : Constant  Value=zeros(3,1)
  Gain : Gain  Gain=pi/180
  Selector1 : Selector  InputPortWidth=Ports.NECK_POS_PORT_SIZE  IndexOptions=Index vector (dialog)  Indices=[1:3]  OutputSizes=1
  Switch : Switch  Criteria=u2 > Threshold
  USE_IMU4EST_BASE1 : Constant  Value=Config.CORRECT_NECK_IMU
  neck position : Outport
  wires:
  neck port/1 -> Gain/1
  USE_IMU4EST_BASE1/1 -> Switch/2
  Switch/1 -> neck position/1
  Gain/1 -> Selector1/1
  Constant/1 -> Switch/3
  Selector1/1 -> Switch/1  "neck pos"

== matlab function Jerk Control/Estimate Contact Forces and Parametrization/From body to Mixed Representation/MATLAB Function ==
  data: w_H_l_sole input double; f_mixed output double; w_H_r_sole input double; f_body input double
function f_mixed = fromBodyToMixedContactForces(w_H_l_sole, w_H_r_sole, f_body)

  f_lFoot = f_body(1:6);
  f_rFoot = f_body(7:12);
  
  f_lFoot = blkdiag(w_H_l_sole(1:3,1:3),w_H_l_sole(1:3,1:3))*f_lFoot;
  f_rFoot = blkdiag(w_H_r_sole(1:3,1:3),w_H_r_sole(1:3,1:3))*f_rFoot;
  
  f_mixed = [f_lFoot; f_rFoot];

end

== matlab function Robot State and References/Internal Coordinator/Base to fixed_link/fixedFoot to base link transform /fromImuToHomogeousTransformFCN ==
  data: imu_H_fixedLink input double; imu_H_fixedLink_0 input double; fixedLink_H_base input double; rpyFromIMU_0 input double; rpyFromIMU input double; neck_pos input double; w_H_b output double; Config parameter double
function w_H_b = getWorldToBaseTransformFCN(imu_H_fixedLink, imu_H_fixedLink_0, fixedLink_H_base, rpyFromIMU_0, rpyFromIMU, neck_pos, Config)

    FILTER_IMU_YAW = Config.FILTER_IMU_YAW;
    
    [w_H_b, wImu_H_base, wImu_H_fixedLink_0] = wbc.worldToBaseTransformWithIMU(imu_H_fixedLink, imu_H_fixedLink_0, fixedLink_H_base, rpyFromIMU_0, rpyFromIMU, FILTER_IMU_YAW);
    
    % Correct head IMU with neck positions (HEAD IMU only)
    if Config.CORRECT_NECK_IMU
        
        wImu_H_wImuAssumingNeckToZero = wbc.correctIMUWithNeckPos(neck_pos);
        wImu_H_base                   = wImu_H_wImuAssumingNeckToZero * wImu_H_base;
        w_H_b                         = wImu_H_fixedLink_0\wImu_H_base;  
    end
end

== matlab function Robot State and References/State Machine Yoga/Compute base to fixed link transform/fixedLFoot to base link transform /fromImuToHomogeousTransformFCN ==
  data: imu_H_fixedLink input double; imu_H_fixedLink_0 input double; fixedLink_H_base input double; rpyFromIMU_0 input double; rpyFromIMU input double; neck_pos input double; w_H_b output double; Config parameter double
function w_H_b = getWorldToBaseTransformFCN(imu_H_fixedLink, imu_H_fixedLink_0, fixedLink_H_base, rpyFromIMU_0, rpyFromIMU, neck_pos, Config)

    FILTER_IMU_YAW = Config.FILTER_IMU_YAW;
    
    [w_H_b, wImu_H_base, wImu_H_fixedLink_0] = wbc.worldToBaseTransformWithIMU(imu_H_fixedLink, imu_H_fixedLink_0, fixedLink_H_base, rpyFromIMU_0, rpyFromIMU, FILTER_IMU_YAW);
    
    % Correct head IMU with neck positions (HEAD IMU only)
    if Config.CORRECT_NECK_IMU
        
        wImu_H_wImuAssumingNeckToZero = wbc.correctIMUWithNeckPos(neck_pos);
        wImu_H_base                   = wImu_H_wImuAssumingNeckToZero * wImu_H_base;
        w_H_b                         = wImu_H_fixedLink_0\wImu_H_base;  
    end
end

== matlab function Robot State and References/Internal Coordinator/Compute State Velocity/Compute Base Velocity ==
  data: J_l_sole input double; J_r_sole input double; feetContactStatus input double; nu_b output double; jointVel input double; Reg parameter double
function nu_b = computeBaseVelocityFCN(J_l_sole, J_r_sole, feetContactStatus, jointVel, Reg)

    pinvDamp_baseVel = Reg.pinvDamp_baseVel;
    
    nu_b = wbc.computeBaseVelocityWithFeetContact(J_l_sole, J_r_sole, feetContactStatus, jointVel, pinvDamp_baseVel);
end

== matlab function Dynamics and Kinematics/Dynamics/Add motors reflected inertia/Add motor reflected inertias ==
  data: M input double; M_with_inertia output double; Config parameter double
function M_with_inertia = addMotorsInertiaFCN(M,Config)

    Gamma = Config.Gamma;
    T     = Config.T;
    I_m   = Config.I_m;
    
    M_with_inertia = wbc.addMotorsReflectedInertia(M,Gamma,T,I_m);
end

== matlab function Robot State and References/State Machine Yoga/Compute State Velocity/Compute Base Velocity ==
  data: J_l_sole input double; J_r_sole input double; feetContactStatus input double; nu_b output double; jointVel input double; Reg parameter double
function nu_b = computeBaseVelocityFCN(J_l_sole, J_r_sole, feetContactStatus, jointVel, Reg)

    pinvDamp_baseVel = Reg.pinvDamp_baseVel;
    
    nu_b = wbc.computeBaseVelocityWithFeetContact(J_l_sole, J_r_sole, feetContactStatus, jointVel, pinvDamp_baseVel);
end

== matlab function Robot State and References/State Machine Yoga/Compute base to fixed link transform/fixedRFoot to base link transform/fromImuToHomogeousTransformFCN ==
  data: imu_H_fixedLink input double; imu_H_fixedLink_0 input double; fixedLink_H_base input double; rpyFromIMU_0 input double; rpyFromIMU input double; neck_pos input double; w_H_b output double; Config parameter double
function w_H_b = getWorldToBaseTransformFCN(imu_H_fixedLink, imu_H_fixedLink_0, fixedLink_H_base, rpyFromIMU_0, rpyFromIMU, neck_pos, Config)

    FILTER_IMU_YAW = Config.FILTER_IMU_YAW;
    
    [w_H_b, wImu_H_base, wImu_H_fixedLink_0] = wbc.worldToBaseTransformWithIMU(imu_H_fixedLink, imu_H_fixedLink_0, fixedLink_H_base, rpyFromIMU_0, rpyFromIMU, FILTER_IMU_YAW);
    
    % Correct head IMU with neck positions (HEAD IMU only)
    if Config.CORRECT_NECK_IMU
        
        wImu_H_wImuAssumingNeckToZero = wbc.correctIMUWithNeckPos(neck_pos);
        wImu_H_base                   = wImu_H_wImuAssumingNeckToZero * wImu_H_base;
        w_H_b                         = wImu_H_fixedLink_0\wImu_H_base;  
    end
end

== matlab function Robot State and References/Internal Coordinator/Reference Generator CoM ==
  data: pos_CoM_0 input double; t input double; references_CoM output double; Config parameter double
function references_CoM = referenceGeneratorCoM_jerkControlFCN(pos_CoM_0, t, Config)
    
    references_CoM = referenceGeneratorCoM_jerkControl(pos_CoM_0, t, Config);
end

== matlab function tauDot Saturation/Saturate Torque Derivative ==
  data: u input double; uSat output double; u_0 input double; tStep input double; uDotMax input double
function uSat = saturateInputDerivativeFCN(u, u_0, tStep, uDotMax)

    uSat = wbc.saturateInputDerivative(u, u_0, tStep, uDotMax);
end

== matlab function Jerk Control/Integrate the Input Contact Forces Param. Derivative/Demux xiDot/Compute Initial Conditions LFoot/Check Previous Foot_in_contact ==
  data: currentFootInContact input double; prevFootBoolean output double
function prevFootBoolean = checkPrevFootInContactFCN(currentFootInContact)

    prevFootBoolean = checkPrevFootInContact(currentFootInContact);
end

== matlab function Robot State and References/State Machine Yoga/stateMachineYogaFCN ==
  data: wrench_rightFoot input double; wrench_leftFoot input double; w_H_b output double; CoM_des output double; qj_des output double; constraints output double; CoM_0 input double; q0 input double; l_sole_CoM input double; r_sole_CoM input double; qj input double; t input double; l_sole_H_b input double; r_sole_H_b input double; Sm parameter double; impedances output double; dampings output double; KPCoM output double; KDCoM output double; Gain parameter double; currentState output double; jointsSmoothingTime output double
function [w_H_b, CoM_des, qj_des, constraints, impedances, dampings, KPCoM, KDCoM, currentState, jointsSmoothingTime] = ...
          stateMachineYogaFCN(wrench_rightFoot, wrench_leftFoot, CoM_0, q0, l_sole_CoM, r_sole_CoM, qj, t, l_sole_H_b, r_sole_H_b, Sm, Gain)
 
    [w_H_b, CoM_des, qj_des, constraints, impedances, dampings, KPCoM, KDCoM, currentState, jointsSmoothingTime] = ...
        stateMachineYoga(CoM_0, q0, l_sole_CoM, r_sole_CoM, qj, t, wrench_rightFoot, wrench_leftFoot, l_sole_H_b, r_sole_H_b, Sm, Gain); 
end

== matlab function emergency stop: joint limits/STOP IF THERE ARE SPIKES IN THE ENCODERS/MATLAB Function ==
  data: u input double; delta_u_max input double; noSpikes output double
function noSpikes = checkSpikes(u, delta_u_max)

     noSpikes = wbc.checkSpikes(u, delta_u_max);
end

== matlab function Jerk Control/Integrate the Input Contact Forces Param. Derivative/Demux xiDot/Compute Initial Conditions RFoot/Check Previous Foot_in_contact ==
  data: currentFootInContact input double; prevFootBoolean output double
function prevFootBoolean = checkPrevFootInContactFCN(currentFootInContact)

    prevFootBoolean = checkPrevFootInContact(currentFootInContact);
end

== matlab function Jerk Control/Integrate the Input Contact Forces Param. Derivative/From Parametrization to Forces/MATLAB Function ==
  data: xi input double; contactForces output double; Config parameter double
function contactForces = fromParametrizationToForcesFCN(xi, Config)
    
    contactForces = fromParametrizationToForces(xi, Config);
end

== matlab function Jerk Control/Momentum Jerk Controller FCN  ==
  data: jointTorques_star output double; LDot_tilde output double; L_tilde output double; intL_tilde output double; xiDes output double; f_des output double; intLTilde_angular input double; nu input double; J_CoM input double; JL input double; JR input double; xCoM input double; w_H_l_sole input double; w_H_r_sole input double; L input double; M input double; h input double; JDotL_nu input double; JDotR_nu input double; x_dx_ddx_dddx_CoM_des input double; gainsPCOM input double; gainsDCOM input double; LEFT_RIGHT_FOOT_IN_CONTACT input double; qj input double; qj_dqj_ddqj_des input double; impedances input double; dampings input double; contactForces_est input double; xi_star input double; xi input double; contactForces_star input double; xiDot_star output double; Config parameter double; Gain parameter double; Reg parameter double
function [jointTorques_star, LDot_tilde, L_tilde, intL_tilde, xiDes, f_des, xiDot_star] = momentumJerkControlYogaFCN(intLTilde_angular, nu, J_CoM, JL, JR, xCoM, w_H_l_sole, w_H_r_sole, L, M, h, JDotL_nu, JDotR_nu, x_dx_ddx_dddx_CoM_des, ...
                                                                                                                     gainsPCOM, gainsDCOM, LEFT_RIGHT_FOOT_IN_CONTACT, qj, qj_dqj_ddqj_des, impedances, dampings, ...
                                                                                                                     contactForces_est, xi_star, xi, contactForces_star,Config, Gain, Reg)
                        
    [jointTorques_star, LDot_tilde, L_tilde, intL_tilde, xiDes, f_des, xiDot_star] = momentumJerkControlYoga(intLTilde_angular, nu, J_CoM, JL, JR, xCoM, w_H_l_sole, w_H_r_sole, L, M, h, JDotL_nu, JDotR_nu, x_dx_ddx_dddx_CoM_des, ...
                                                                                                             gainsPCOM, gainsDCOM, LEFT_RIGHT_FOOT_IN_CONTACT, qj, qj_dqj_ddqj_des, impedances, dampings, ...
                                                                                                             contactForces_est, xi_star, xi, contactForces_star, Config, Gain, Reg);                   
end

== matlab function emergency stop: joint limits/STOP IF JOINTS HIT THE LIMITS/MATLAB Function ==
  data: umin input double; umax input double; u input double; inRange output double; tol input double
function inRange = checkRangeFCN(umin, umax, u, tol)

     inRange = wbc.checkRange(umin, umax, u, tol);
end

== matlab function Jerk Control/Integrate the Input Contact Forces Param. Derivative/From Parametrization to Forces/MATLAB Function1 ==
  data: xi input double; contactForces output double; Config parameter double
function contactForces = fromParametrizationToForcesFCN(xi, Config)
    
    contactForces = fromParametrizationToForces(xi, Config);
end

== matlab function Jerk Control/Integrate the Input Contact Forces Param. Derivative/Demux xiDot/MATLAB Function1 ==
  data: contactForces input double; xi output double; Config parameter double
function xi = fromForcesToParametrizationFCN(contactForces, Config)
    
    xi = fromForcesToParametrization(contactForces, Config);
end

== matlab function Jerk Control/Integrate the Input Contact Forces Param. Derivative/Demux xiDot/MATLAB Function2 ==
  data: contactForces input double; xi output double; Config parameter double
function xi = fromForcesToParametrizationFCN(contactForces, Config)
    
    xi = fromForcesToParametrization(contactForces, Config);
end

== matlab function Jerk Control/Integrate the Input Contact Forces Param. Derivative/deadZone/MATLAB Function ==
  data: u input double; y output double; thr input double
function y = deadZoneFCN(u, thr)

    y = wbc.deadZone(u, thr);
end

== matlab function Jerk Control/Estimate Contact Forces and Parametrization/Get Parametrization from Forces/MATLAB Function1 ==
  data: contactForces input double; xi output double; Config parameter double
function xi = fromForcesToParametrizationFCN(contactForces, Config)
    
    xi = fromForcesToParametrization(contactForces, Config);
end

== matlab function Jerk Control/Compute joint torques (motor reflected inertia)/(transpose(T*Gamma))^{-1}*I_m*(T*Gamma)^{-1}1 ==
  data: reflectedInertia output double; Config parameter double
function reflectedInertia  = computeMotorsInertiaFCN(Config)
    
    Gamma = Config.Gamma;
    T     = Config.T;
    I_m   = Config.I_m;
    
    reflectedInertia = wbc.computeMotorsReflectedInertia(Gamma,T,I_m);
end

== matlab function Jerk Control/Estimate Contact Forces and Parametrization/Get Parametrization from Forces/MATLAB Function2 ==
  data: contactForces input double; xi output double; Config parameter double
function xi = fromForcesToParametrizationFCN(contactForces, Config)
    
    xi = fromForcesToParametrization(contactForces, Config);
end

== matlab function Jerk Control/Compute angular momentum integral error (YOGA)/Get Equivalent Base Velocity ==
  data: J_l_sole input double; J_r_sole input double; feetContactStatus input double; jointPos_err input double; baseVel_equivalent output double; Reg parameter double
function baseVel_equivalent = getEquivalentBaseVel_FCN(J_l_sole, J_r_sole, feetContactStatus, jointPos_err, Reg)

    if feetContactStatus(1) == 1
    
        pinvJb             = (J_l_sole(:,1:6)'*J_l_sole(:,1:6) + Reg.pinvDamp_baseVel*eye(6))\J_l_sole(:,1:6)';
        baseVel_equivalent = -pinvJb*J_l_sole(:,7:end)*jointPos_err;
    else
        pinvJb             = (J_r_sole(:,1:6)'*J_r_sole(:,1:6) + Reg.pinvDamp_baseVel*eye(6))\J_r_sole(:,1:6)';
        baseVel_equivalent = -pinvJb*J_r_sole(:,7:end)*jointPos_err;
    end
end

== matlab function Jerk Control/Compute angular momentum integral error (YOGA)/Select base to world transform ==
  data: state input double; booleanState output double
function booleanState = footOnGround(state)

    % output: a boolean variable whose value is 1 if the foot on ground is left
    % foot, and 0 if the foot on ground is the right foot. If both feet are on
    % ground, the variable is setted to 1.

    % states in which right foot is on ground: 9,10,11,12 (HARD CODED)
    booleanState = 1;

    if state == 9 || state == 10 || state == 11 || state == 12

        booleanState = 0;
    end
end

== matlab function Jerk Control/Estimate Contact Forces and Parametrization/Contact Forces From Dynamics ==
  data: tau input double; JL input double; JR input double; JDotL_nu input double; JDotR_nu input double; M input double; h input double; LEFT_RIGHT_FOOT_IN_CONTACT input double; f_dynamics output double
function f_dynamics = estimateContactForcesFromDynamicsFCN(tau, JL, JR, JDotL_nu, JDotR_nu, M, h, LEFT_RIGHT_FOOT_IN_CONTACT)
                                        
    f_dynamics = estimateContactForcesFromDynamics(tau, JL, JR, JDotL_nu, JDotR_nu, M, h, LEFT_RIGHT_FOOT_IN_CONTACT);
end
